simulink model "Feedback"  (R2021a)
settings: Solver=VariableStepAuto  StartTime=0.0  StopTime=10.0  RelTol=1e-3
values from neighbouring files (symbols this model uses):
  A = [0 0 1 0;0 0 0 1;1 0 0 -20;4.998 -70 -49.98 0]    [Controlib.m]    (also in Observ.m = [0 0 1 0; 0 0 0 1;1 0 0 -20;4.998 -70 -49.98 0]; Opp.m = double(subs(jac,[x1,x2,x3,x4],[op1,op2,op3,op4])); Stabili.m = [0 0 1 0; 0 0 0 1;1 0 0 -20;4.998 -70 -49.98 0]; lyaptesting.m = [0 0 1 0;0 0 0 1;1 0 0 -20;5 -70 -50 0])
  B = [0 0;0 0;F/7 0;0 M/2]    [Controlib.m]    (also in Linearization.m; Observ.m = [0 0;0 0 ;F/7 0 ; 0 M/2]; Opp.m; Stabili.m = [0 0;0 0; F/7 0; 0 M/2])
  C = [1 0 0 0 ;0 1 0 0]    [Controlib.m]    (also in Linearization.m = [1 0 0 0;0 1 0 0]; Observ.m = [1 0 0 0;0 1 0 0]; Opp.m = [1 0 0 0;0 1 0 0]; Stabili.m = [1 0 0 0; 0 1 0 0])
  K = place(A,B,PR)    [Poleplace.m]
settings Model: Creator=bahet  LastModifiedBy=bahet

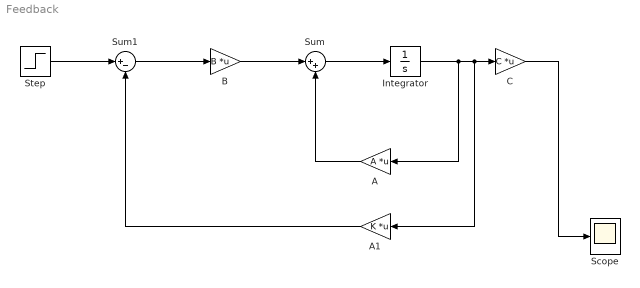
== system Feedback ==
  A : Gain  Gain=A  Multiplication=Matrix(K*u)
  A1 : Gain  Gain=K  Multiplication=Matrix(K*u)
  B : Gain  Gain=B  Multiplication=Matrix(K*u)
  C : Gain  Gain=C  Multiplication=Matrix(K*u)
  Integrator : Integrator
  Scope : Scope
  Step : Step  Time=0  After=[1;1]  SampleTime=0
  Sum : Sum  Inputs=|++
  Sum1 : Sum  Inputs=|+-
  wires:
  Integrator/1 -> A/1, A1/1, C/1
  A1/1 -> Sum1/2
  Step/1 -> Sum1/1
  Sum/1 -> Integrator/1
  B/1 -> Sum/1
  Sum1/1 -> B/1
  A/1 -> Sum/2
  C/1 -> Scope/1
